simulink model "DTC"  (R2021a)
settings: Solver=ode4  StartTime=0.0  StopTime=10  FixedStep=1e-4  MaxStep=1e-3  RelTol=1e-3  EnableMultiTasking=on
model workspace (MAT data in the model file):
  hh = 1
values from neighbouring files (symbols this model uses):
  mm = [0	0 ... (first row only)    [tab1.m]
  p = 2    [Parametres.m]
libraries: simulink x3
settings Model: Creator=Prox Info  LastModifiedBy=Mohanad Bahar
settings SolverCC: AlgebraicLoopSolver=TrustRegion
settings DataIOCC: LimitDataPoints=on  SaveFormat=Array  SignalLoggingSaveFormat=ModelDataLogs  ReturnWorkspaceOutputs=off  SignalLoggingName=sigsOut
settings OptimizationCC: ExpressionDepthLimit=2147483647  LifeSpan=inf
settings DebuggingCC: SaveWithParameterizedLinksMsg=none  UnderspecifiedInitializationDetection=Classic  MergeDetectMultiDrivingBlocksExec=none  SignalResolutionControl=TryResolveAllWithWarning  MultiTaskDSMMsg=warning  MultiTaskCondExecSysMsg=none  FcnCallInpInsideContextMsg=warning  StateNameClashWarn=warning  SFUnexpectedBacktrackingDiag=warning  SFNoUnconditionalDefaultTransitionDiag=warning  SFExecutionAtInitializationDiag=none  SFMachineParentedDataDiag=warning  ArithmeticOperatorsInVariantConditions=warning
settings HardwareCC: ProdBitPerPointer=32  ProdBitPerSizeT=32  ProdBitPerPtrDiffT=32  ProdLargestAtomicFloat=None  ProdIntDivRoundTo=Undefined  ProdEndianess=Unspecified  ProdWordSize=32  ProdHWDeviceType=32-bit Generic  TargetUnknown=on
settings ModelReferenceCC: PropagateSignalLabelsOutOfModel=off
settings SFSimCC: SimUseLocalCustomCode=off  CustomCodeUndefinedFunction=UseInterfaceOnly
settings RTWCC: RTWUseLocalCustomCode=off
settings CodeAppCC: StateflowObjectComments=on
settings GRTTargetCC: TargetLangStandard=C89/C90 (ANSI)  CombineOutputUpdateFcns=off  GRTInterface=on
settings ConfigComp: CovMetricSettings=dw  CovSaveCumulativeToWorkspaceVar=on  CovSaveSingleToWorkspaceVar=on  CovExternalEMLEnable=off

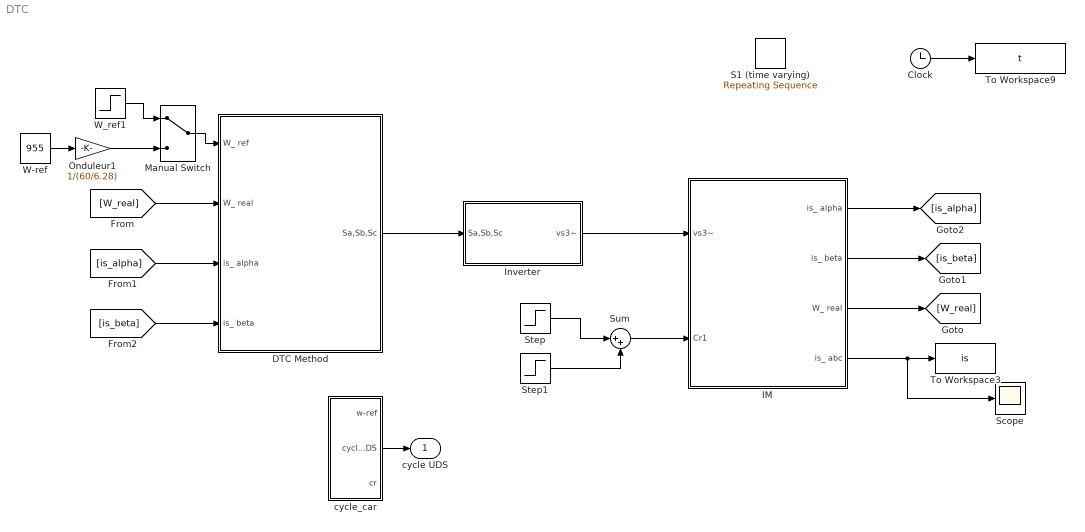
== system DTC ==
  Clock : Clock
  DTC Method : Subsystem
  IM : Subsystem  mask{Rs=1.2, Rr=1.8, Ls=0.1558, Lr=0.1568, M=0.15, p=2, J=0.07, f=0}
      mask prompts: Rs "Rs="; Rr "Rr="; Ls "Ls="; Lr "Lr="; M "M="; p "p="; J "J="; f "f="
  Inverter : Subsystem
  Manual Switch : ManualSwitch
  Onduleur1 : Gain  Gain=1/(60/6.28)  SaturateOnIntegerOverflow=on  OutDataTypeStr=Inherit: Same as input  ParamDataTypeStr=Inherit: Same as input
  S1 (time varying) : simulink/Sources/Repeating Sequence  rep_seq_t=[1 2 3]  rep_seq_y=[1 0.5 1.2 ]
  Scope : Scope
  Step : Step  Time=3  After=20  SampleTime=0
  Step1 : Step  Time=7  After=-20  SampleTime=0
  Sum : Sum  Inputs=|++
  To Workspace3 : ToWorkspace  VariableName=is  SampleTime=-1
  To Workspace9 : ToWorkspace  VariableName=t  SampleTime=-1
  W-ref : Constant  Value=955
  W_ref1 : Step  Time=4  Before=100  After=-100  SampleTime=0
  cycle_car : Subsystem
  cycle UDS : Outport
  wires:
  Clock/1 -> To Workspace9/1
  IM/4(is_ abc) -> Scope/1, To Workspace3/1
  IM/3(W_ real) -> [W_real]
  [W_real] -> DTC Method/2(W_ real)
  IM/2(is_ beta) -> [is_beta]
  IM/1(is_ alpha) -> [is_alpha]
  [is_alpha] -> DTC Method/3(is_ alpha)
  [is_beta] -> DTC Method/4(is_ beta)
  DTC Method/1("Sa,Sb,Sc ") -> Inverter/1("Sa,Sb,Sc ")
  Inverter/1(vs3~) -> IM/1(vs3~)
  cycle_car/2(cycle UDS) -> cycle UDS/1
  W-ref/1 -> Onduleur1/1
  Step/1 -> Sum/1
  Step1/1 -> Sum/2
  Onduleur1/1 -> Manual Switch/2
  W_ref1/1 -> Manual Switch/1
  Manual Switch/1 -> DTC Method/1(W_ ref)
  Sum/1 -> IM/2(Cr1)

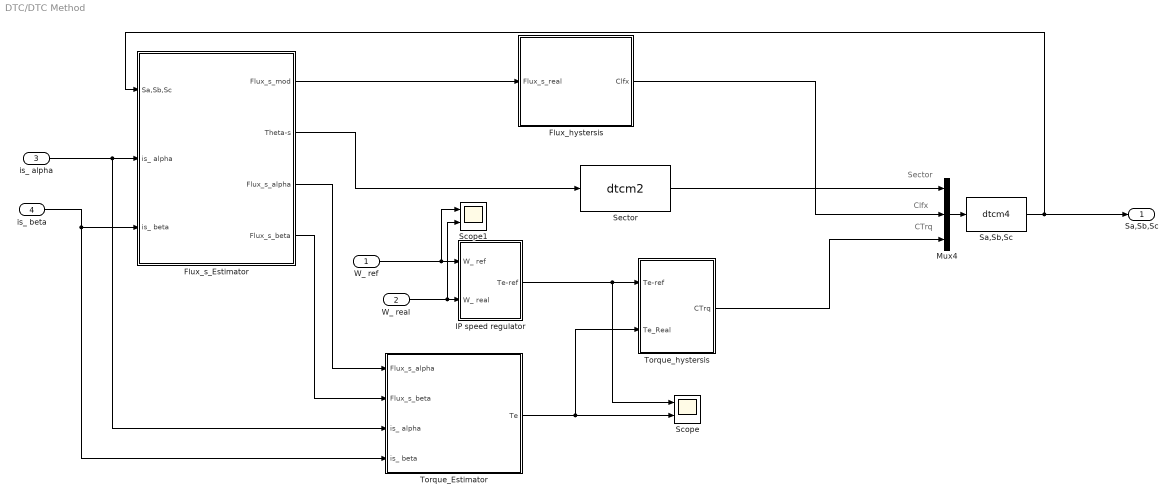
== system DTC/DTC Method ==
  note: CTrq
  note: Sector
  note: Clfx
  W_ ref : Inport
  W_ real : Inport  Port=2
  is_ alpha : Inport  Port=3
  is_ beta : Inport  Port=4
  Flux_hystersis : Subsystem
  Flux_s_Estimator : Subsystem  mask{Rs=1.2, p=2}
  IP speed regulator : Subsystem
  Mux4 : Mux  Inputs=3
  Sa,Sb,Sc : MATLABFcn  MATLABFcn=dtcm4  OutputDimensions=3
  Scope : Scope  NumInputPorts=2
  Scope1 : Scope  NumInputPorts=2
  Sector : MATLABFcn  MATLABFcn=dtcm2  OutputDimensions=1
  Torque_Estimator : Subsystem
  Torque_hystersis : Subsystem
  "Sa,Sb,Sc " : Outport
  wires:
  Mux4/1 -> Sa,Sb,Sc/1
  Sector/1 -> Mux4/1
  Sa,Sb,Sc/1 -> Flux_s_Estimator/1(Sa,Sb,Sc), "Sa,Sb,Sc "/1
  W_ real/1 -> Scope1/2, IP speed regulator/2(W_ real)
  Flux_s_Estimator/3(Flux_s_alpha) -> Torque_Estimator/1(Flux_s_alpha)
  Flux_s_Estimator/4(Flux_s_beta) -> Torque_Estimator/2(Flux_s_beta)
  is_ alpha/1 -> Torque_Estimator/3(is_ alpha), Flux_s_Estimator/2(is_ alpha)
  is_ beta/1 -> Torque_Estimator/4(is_ beta), Flux_s_Estimator/3(is_ beta)
  Flux_s_Estimator/2("Theta-s ") -> Sector/1
  Flux_s_Estimator/1(Flux_s_mod) -> Flux_hystersis/1(Flux_s_real)
  Flux_hystersis/1(Clfx) -> Mux4/2
  IP speed regulator/1(Te-ref) -> Scope/1, Torque_hystersis/1(Te-ref)
  Torque_Estimator/1(Te) -> Torque_hystersis/2(Te_Real), Scope/2
  Torque_hystersis/1(CTrq) -> Mux4/3
  W_ ref/1 -> Scope1/1, IP speed regulator/1(W_ ref)

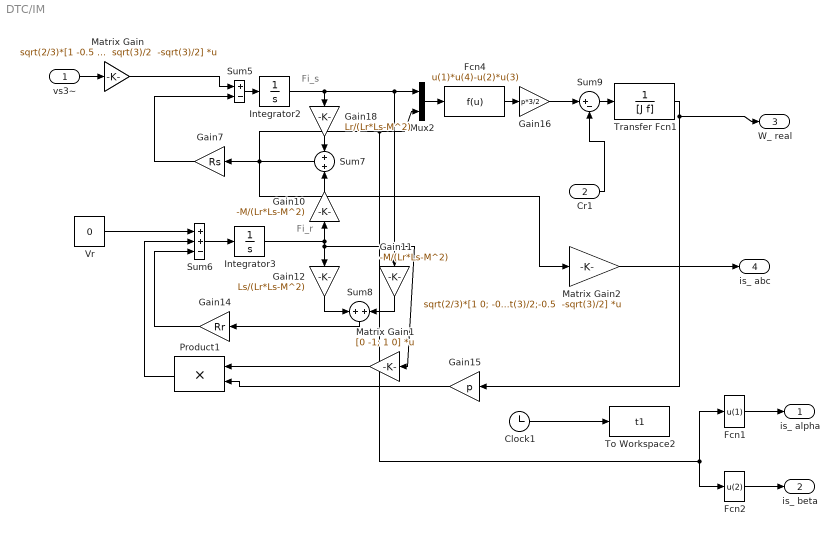
== system DTC/IM ==
  note: Fi_s
  note: Fi_r
  vs3~ : Inport
  Cr1 : Inport  Port=2
  Clock1 : Clock
  Fcn1 : Fcn  Expr=u(1)
  Fcn2 : Fcn  Expr=u(2)
  Fcn4 : Fcn  Expr=u(1)*u(4)-u(2)*u(3)
  Gain10 : Gain  Gain=-M/(Lr*Ls-M^2)  SaturateOnIntegerOverflow=on  OutDataTypeStr=Inherit: Same as input  ParamDataTypeStr=Inherit: Same as input
  Gain11 : Gain  Gain=-M/(Lr*Ls-M^2)  SaturateOnIntegerOverflow=on  OutDataTypeStr=Inherit: Same as input  ParamDataTypeStr=Inherit: Same as input
  Gain12 : Gain  Gain=Ls/(Lr*Ls-M^2)  SaturateOnIntegerOverflow=on  OutDataTypeStr=Inherit: Same as input  ParamDataTypeStr=Inherit: Same as input
  Gain14 : Gain  Gain=Rr  SaturateOnIntegerOverflow=on  OutDataTypeStr=Inherit: Same as input  ParamDataTypeStr=Inherit: Same as input
  Gain15 : Gain  Gain=p  SaturateOnIntegerOverflow=on  OutDataTypeStr=Inherit: Same as input  ParamDataTypeStr=Inherit: Same as input
  Gain16 : Gain  Gain=p*3/2  SaturateOnIntegerOverflow=on  OutDataTypeStr=Inherit: Same as input  ParamDataTypeStr=Inherit: Same as input
  Gain18 : Gain  Gain=Lr/(Lr*Ls-M^2)  SaturateOnIntegerOverflow=on  OutDataTypeStr=Inherit: Same as input  ParamDataTypeStr=Inherit: Same as input
  Gain7 : Gain  Gain=Rs  SaturateOnIntegerOverflow=on  OutDataTypeStr=Inherit: Same as input  ParamDataTypeStr=Inherit: Same as input
  Integrator2 : Integrator
  Integrator3 : Integrator
  Matrix Gain : Gain  Gain="sqrt(2/3)*[1 -0.5  -0.5;  0  sqrt(3)/2  -sqrt(3)/2]"  Multiplication=Matrix(K*u)  SaturateOnIntegerOverflow=on  OutDataTypeStr=Inherit: Same as input  ParamDataTypeStr=Inherit: Same as input
  Matrix Gain1 : Gain  Gain=[0 -1; 1 0]  Multiplication=Matrix(K*u)  SaturateOnIntegerOverflow=on  OutDataTypeStr=Inherit: Same as input  ParamDataTypeStr=Inherit: Same as input
  Matrix Gain2 : Gain  Gain="sqrt(2/3)*[1 0; -0.5  sqrt(3)/2;-0.5  -sqrt(3)/2]"  Multiplication=Matrix(K*u)  SaturateOnIntegerOverflow=on  OutDataTypeStr=Inherit: Same as input  ParamDataTypeStr=Inherit: Same as input
  Mux2 : Mux  Inputs=2
  Product1 : Product  SaturateOnIntegerOverflow=on  OutDataTypeStr=Inherit: Same as first input
  Sum5 : Sum  Inputs=+-  SaturateOnIntegerOverflow=on
  Sum6 : Sum  Inputs=++-  SaturateOnIntegerOverflow=on
  Sum7 : Sum  SaturateOnIntegerOverflow=on
  Sum8 : Sum  SaturateOnIntegerOverflow=on
  Sum9 : Sum  Inputs=|+-  SaturateOnIntegerOverflow=on
  To Workspace2 : ToWorkspace  VariableName=t1  SampleTime=-1
  Transfer Fcn1 : TransferFcn  Denominator=[J f]
  Vr : Constant  Value=0
  is_ alpha : Outport
  is_ beta : Outport  Port=2
  W_ real : Outport  Port=3
  is_ abc : Outport  Port=4
  wires:
  Sum6/1 -> Integrator3/1
  Sum5/1 -> Integrator2/1
  Gain7/1 -> Sum5/2
  Integrator2/1 -> Mux2/1, Gain11/1, Gain18/1
  Gain18/1 -> Sum7/1
  Sum7/1 -> Gain7/1, Mux2/2, Fcn1/1, Fcn2/1, Matrix Gain2/1
  Gain10/1 -> Sum7/2
  Integrator3/1 -> Matrix Gain1/1, Gain12/1, Gain10/1
  Gain11/1 -> Sum8/2
  Gain12/1 -> Sum8/1
  Sum8/1 -> Gain14/1
  Gain14/1 -> Sum6/3
  Matrix Gain1/1 -> Product1/1
  Product1/1 -> Sum6/2
  Mux2/1 -> Fcn4/1
  Fcn4/1 -> Gain16/1
  Gain16/1 -> Sum9/1
  Sum9/1 -> Transfer Fcn1/1
  Transfer Fcn1/1 -> Gain15/1, W_ real/1
  Gain15/1 -> Product1/2
  Clock1/1 -> To Workspace2/1
  Vr/1 -> Sum6/1
  Cr1/1 -> Sum9/2
  Fcn1/1 -> is_ alpha/1
  Fcn2/1 -> is_ beta/1
  Matrix Gain/1 -> Sum5/1
  vs3~/1 -> Matrix Gain/1
  Matrix Gain2/1 -> is_ abc/1

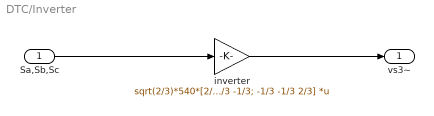
== system DTC/Inverter ==
  "Sa,Sb,Sc " : Inport
  inverter : Gain  Gain=sqrt(2/3)*540*[2/3 -1/3 -1/3;-1/3 2/3 -1/3; -1/3 -1/3 2/3]  Multiplication=Matrix(K*u)  SaturateOnIntegerOverflow=on  OutDataTypeStr=Inherit: Same as input  ParamDataTypeStr=Inherit: Same as input
  vs3~ : Outport
  wires:
  "Sa,Sb,Sc "/1 -> inverter/1
  inverter/1 -> vs3~/1

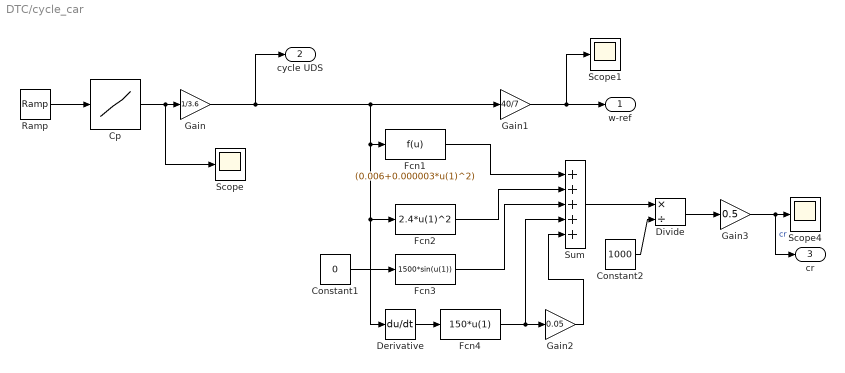
== system DTC/cycle_car ==
  Constant1 : Constant  Value=0
  Constant2 : Constant  Value=1000
  Cp : Lookup  InputValues=mm(:,1)  Table=mm(:,2)  SaturateOnIntegerOverflow=on
  Derivative : Derivative
  Divide : Product  Inputs=*/
  Fcn1 : Fcn  Expr=(0.006+0.000003*u(1)^2)
  Fcn2 : Fcn  Expr=2.4*u(1)^2
  Fcn3 : Fcn  Expr=1500*sin(u(1))
  Fcn4 : Fcn  Expr=150*u(1)
  Gain : Gain  Gain=1/3.6
  Gain1 : Gain  Gain=40/7
  Gain2 : Gain  Gain=0.05
  Gain3 : Gain  Gain=0.5
  Ramp : simulink/Sources/Ramp  slope=140  start=0  InitialOutput=0
  Scope : Scope
  Scope1 : Scope
  Scope4 : Scope
  Sum : Sum  Inputs=+++++
  w-ref : Outport
  cycle UDS : Outport  Port=2
  cr : Outport  Port=3
  wires:
  Divide/1 -> Gain3/1
  Cp/1 -> Scope/1, Gain/1
  Constant1/1 -> Fcn3/1
  Fcn4/1 -> Sum/4, Gain2/1
  Constant2/1 -> Divide/2
  Sum/1 -> Divide/1
  Fcn1/1 -> Sum/1
  Gain/1 -> cycle UDS/1, Fcn1/1, Fcn2/1, Derivative/1, Gain1/1
  Fcn2/1 -> Sum/2
  Gain1/1 -> w-ref/1, Scope1/1
  Fcn3/1 -> Sum/3
  Ramp/1 -> Cp/1
  Gain2/1 -> Sum/5
  Derivative/1 -> Fcn4/1
  Gain3/1 -> cr/1, Scope4/1  "cr"

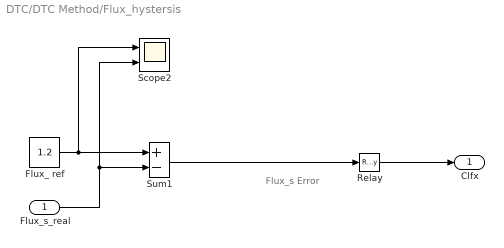
== system DTC/DTC Method/Flux_hystersis ==
  note: Flux_s Error
  Flux_s_real : Inport
  Flux_ ref : Constant  Value=1.2
  Relay : Relay  OffSwitchValue=-eps
  Scope2 : Scope  NumInputPorts=2
  Sum1 : Sum  Inputs=+-  SaturateOnIntegerOverflow=on
  Clfx : Outport
  wires:
  Flux_ ref/1 -> Scope2/1, Sum1/1
  Sum1/1 -> Relay/1
  Relay/1 -> Clfx/1
  Flux_s_real/1 -> Scope2/2, Sum1/2

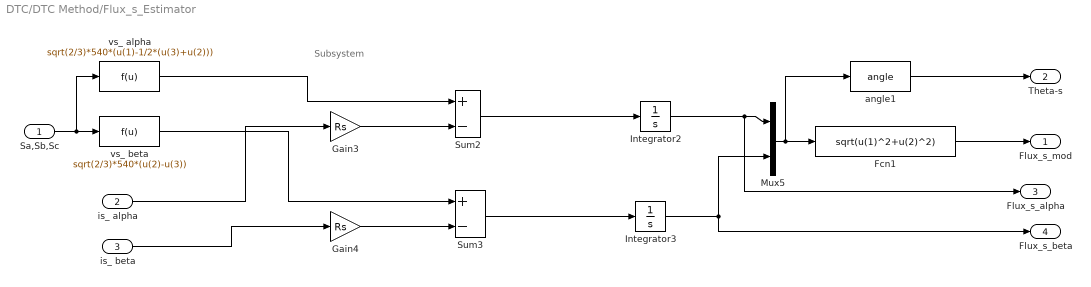
== system DTC/DTC Method/Flux_s_Estimator ==
  note: Subsystem
  Sa,Sb,Sc : Inport
  is_ alpha : Inport  Port=2
  is_ beta : Inport  Port=3
  Fcn1 : Fcn  Expr=sqrt(u(1)^2+u(2)^2)
  Gain3 : Gain  Gain=Rs  SaturateOnIntegerOverflow=on  OutDataTypeStr=Inherit: Same as input  ParamDataTypeStr=Inherit: Same as input
  Gain4 : Gain  Gain=Rs  SaturateOnIntegerOverflow=on  OutDataTypeStr=Inherit: Same as input  ParamDataTypeStr=Inherit: Same as input
  Integrator2 : Integrator
  Integrator3 : Integrator
  Mux5 : Mux  Inputs=2
  Sum2 : Sum  Inputs=+-  SaturateOnIntegerOverflow=on
  Sum3 : Sum  Inputs=+-  SaturateOnIntegerOverflow=on
  angle1 : MATLABFcn  MATLABFcn=angle  OutputDimensions=1
  vs_ alpha : Fcn  Expr=sqrt(2/3)*540*(u(1)-1/2*(u(3)+u(2)))
  vs_ beta : Fcn  Expr=sqrt(2/3)*540*(u(2)-u(3))
  Flux_s_mod : Outport
  "Theta-s " : Outport  Port=2
  Flux_s_alpha : Outport  Port=3
  Flux_s_beta : Outport  Port=4
  wires:
  Sa,Sb,Sc/1 -> vs_ alpha/1, vs_ beta/1
  angle1/1 -> "Theta-s "/1
  Fcn1/1 -> Flux_s_mod/1
  Integrator2/1 -> Flux_s_alpha/1, Mux5/1
  Integrator3/1 -> Flux_s_beta/1, Mux5/2
  vs_ alpha/1 -> Sum2/1
  vs_ beta/1 -> Sum3/1
  Sum3/1 -> Integrator3/1
  is_ alpha/1 -> Gain3/1
  Mux5/1 -> angle1/1, Fcn1/1
  Gain4/1 -> Sum3/2
  is_ beta/1 -> Gain4/1
  Sum2/1 -> Integrator2/1
  Gain3/1 -> Sum2/2

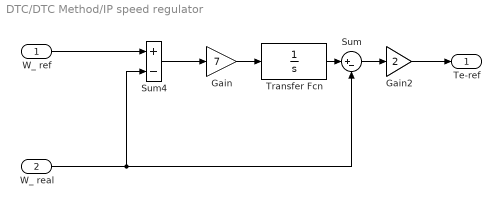
== system DTC/DTC Method/IP speed regulator ==
  W_ ref : Inport
  W_ real : Inport  Port=2
  Gain : Gain  Gain=7  SaturateOnIntegerOverflow=on  OutDataTypeStr=Inherit: Same as input  ParamDataTypeStr=Inherit: Same as input
  Gain2 : Gain  Gain=2  SaturateOnIntegerOverflow=on  OutDataTypeStr=Inherit: Same as input  ParamDataTypeStr=Inherit: Same as input
  Sum : Sum  Inputs=|+-  InputSameDT=on  SaturateOnIntegerOverflow=on  OutDataTypeStr=Inherit: Same as first input
  Sum4 : Sum  Inputs=+-  SaturateOnIntegerOverflow=on
  Transfer Fcn : TransferFcn  Denominator=[1 0]
  Te-ref : Outport
  wires:
  Gain/1 -> Transfer Fcn/1
  Transfer Fcn/1 -> Sum/1
  Gain2/1 -> Te-ref/1
  Sum/1 -> Gain2/1
  W_ ref/1 -> Sum4/1
  W_ real/1 -> Sum4/2, Sum/2
  Sum4/1 -> Gain/1

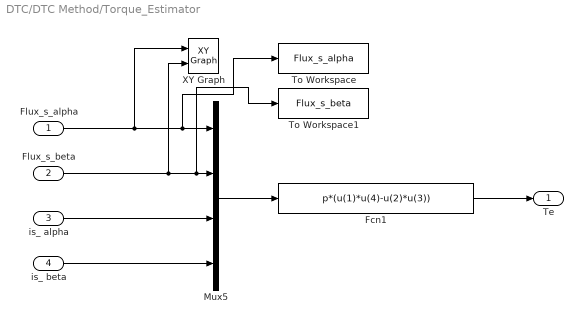
== system DTC/DTC Method/Torque_Estimator ==
  Flux_s_alpha : Inport
  Flux_s_beta : Inport  Port=2
  is_ alpha : Inport  Port=3
  is_ beta : Inport  Port=4
  Fcn1 : Fcn  Expr=p*(u(1)*u(4)-u(2)*u(3))
  Mux5 : Mux
  To Workspace : ToWorkspace  VariableName=Flux_s_alpha  SampleTime=-1
  To Workspace1 : ToWorkspace  VariableName=Flux_s_beta  SampleTime=-1
  XY Graph : simulink/Sinks/XY Graph  xmin=-1.5  xmax=1.5  ymin=-1.5  ymax=1.5  st=-1
  Te : Outport
  wires:
  Fcn1/1 -> Te/1
  is_ beta/1 -> Mux5/4
  Mux5/1 -> Fcn1/1
  is_ alpha/1 -> Mux5/3
  Flux_s_alpha/1 -> XY Graph/1, To Workspace/1, Mux5/1
  Flux_s_beta/1 -> XY Graph/2, To Workspace1/1, Mux5/2

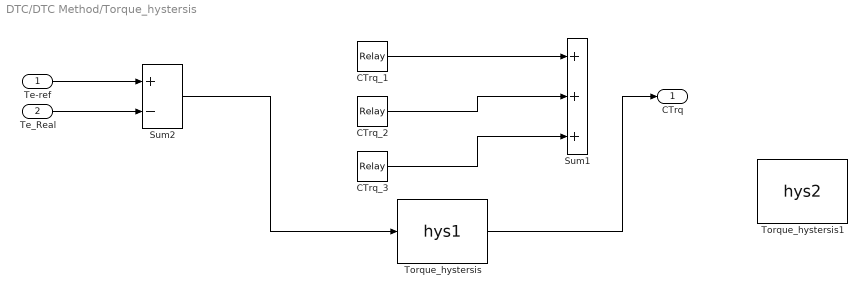
== system DTC/DTC Method/Torque_hystersis ==
  Te-ref : Inport
  Te_Real : Inport  Port=2
  CTrq_1 : Relay  OnSwitchValue=2*eps  OnOutputValue=2  OffOutputValue=1
  CTrq_2 : Relay  OffSwitchValue=-eps  OffOutputValue=-1
  CTrq_3 : Relay  OnSwitchValue=-eps  OffSwitchValue=-2*eps  OnOutputValue=-1  OffOutputValue=-2
  Sum1 : Sum  Inputs=+++
  Sum2 : Sum  Inputs=+-  SaturateOnIntegerOverflow=on
  Torque_hystersis : MATLABFcn  MATLABFcn=hys1  OutputDimensions=1
  Torque_hystersis1 : MATLABFcn  MATLABFcn=hys2  OutputDimensions=1
  CTrq : Outport
  wires:
  Te_Real/1 -> Sum2/2
  Te-ref/1 -> Sum2/1
  CTrq_1/1 -> Sum1/1
  CTrq_3/1 -> Sum1/3
  CTrq_2/1 -> Sum1/2
  Sum2/1 -> Torque_hystersis/1
  Torque_hystersis/1 -> CTrq/1
